simulink model "FForLoop"  (R2018b)
settings: Solver=VariableStepAuto  StartTime=0.0  StopTime=10.0  RelTol=1e-3
settings Model: Creator=Mostafa  LastModifiedBy=Mostafa

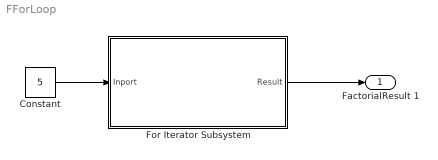
== system FForLoop ==
  Constant : Constant  Value=5
  For Iterator Subsystem : Subsystem  TreatAsAtomicUnit=on
  FactorialResult 1 : Outport
  wires:
  Constant/1 -> For Iterator Subsystem/1(Inport)
  For Iterator Subsystem/1("Result ") -> FactorialResult 1/1

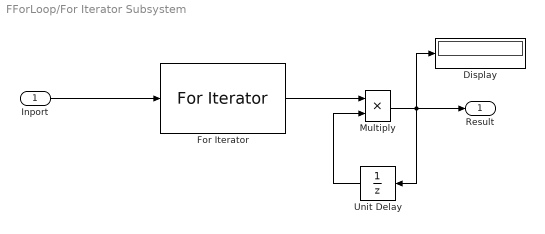
== system FForLoop/For Iterator Subsystem ==
  Inport : Inport
  Display : Display
  For Iterator : ForIterator  ResetStates=reset  IterationSource=external  IterationVariableDataType=int8
  Multiply : Product  OutDataTypeStr=uint8
  Unit Delay : UnitDelay  InitialCondition=1  SampleTime=-1
  "Result " : Outport
  wires:
  Inport/1 -> For Iterator/1
  Unit Delay/1 -> Multiply/2
  Multiply/1 -> Display/1, Unit Delay/1, "Result "/1
  For Iterator/1 -> Multiply/1
